simulink model "EX5_zadanie3"  (R2023b)
settings: Solver=FixedStepDiscrete  StartTime=0.0  StopTime=0  RelTol=1e-3
libraries: CPOiS_SourcesSinks x3, CPOiS_LinearTransforms x2, simulink_extras x1, CPOiS_DataManipulation x1, CPOiS_DataManipulation_DataTypeConversion x1
settings Model: Creator=alyskawa  LastModifiedBy=alyskawa

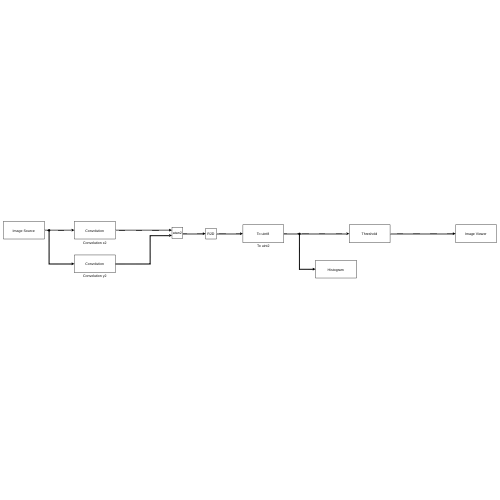
[thumbnail: Simulink's stored preview of the top-level diagram]
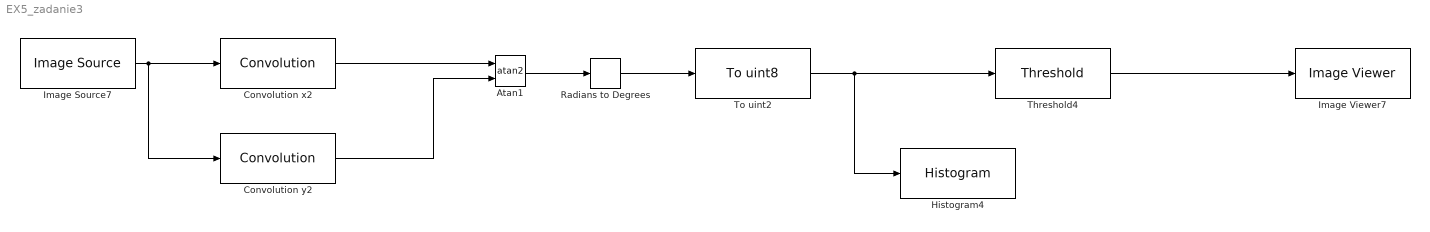
== system EX5_zadanie3 ==
  Atan1 : Trigonometry  Operator=atan2
  Convolution x2 : CPOiS_LinearTransforms/Convolution  ConvolutionMatrix=[-1,0,1;-2,0,2;-1,0,1]
      settings: SourceProductName=CPOiS - Digital image and signal processing
  Convolution y2 : CPOiS_LinearTransforms/Convolution  ConvolutionMatrix=[-1,-2,-1;0,0,0;1,2,1]
      settings: SourceProductName=CPOiS - Digital image and signal processing
  Histogram4 : CPOiS_SourcesSinks/Histogram
      settings: SourceProductName=CPOiS - Digital image and signal processing
  Image Source7 : CPOiS_SourcesSinks/Image Source  FileSelection=coins.png
      settings: SourceProductName=CPOiS - Digital image and signal processing
  Image Viewer7 : CPOiS_SourcesSinks/Image Viewer
      settings: SourceProductName=CPOiS - Digital image and signal processing
  Radians to Degrees : simulink_extras/Transformations/Radians to Degrees
  Threshold4 : CPOiS_DataManipulation/Threshold  Threshold=15
      settings: SourceProductName=CPOiS - Digital image and signal processing
  To uint2 : CPOiS_DataManipulation_DataTypeConversion/To uint8
      settings: SourceProductName=CPOiS - Digital image and signal processing
  wires:
  Radians to Degrees/1 -> To uint2/1
  Threshold4/1 -> Image Viewer7/1
  To uint2/1 -> Histogram4/1, Threshold4/1
  Convolution x2/1 -> Atan1/1
  Convolution y2/1 -> Atan1/2
  Image Source7/1 -> Convolution y2/1, Convolution x2/1
  Atan1/1 -> Radians to Degrees/1
